simulink model "trimLiepke"  (R2021a)
settings: Solver=ode45  StartTime=0.0  StopTime=1000  RelTol=1e-3  EnableMultiTasking=on
undefined symbols (not defined in the file or in its folder): alpha_matrix, alphai, alt_matrix, b, beta, cbar, CD_0, CD_alpha, CD_de, CD_ih, CD_q, CL_0, Cl_0, CL_alpha, Cl_beta, Cl_da, CL_de, Cl_dr, CL_ih, Cl_p, CL_q, Cl_r, cla_matrix, clb_matrix, clp_matrix, clq_matrix, clr_matrix, Cm_0, Cm_alpha, Cm_de, Cm_ih, Cm_q, cma_matrix, cmq_matrix, Cn_0, Cn_beta, Cn_da, Cn_dr, Cn_p, Cn_r, cnb_matrix, cnp_matrix, cnr_matrix, CY_0, CY_beta, CY_da, CY_dr, CY_p, CY_r, cyb_matrix, cyp_matrix, H, Ix, Iy, Iz, Jxy, Jxz, Jyz, m, mach_matrix ... (+10)
libraries: airlib x3
(part 1 of 2)
settings Model: Creator=matt  LastModifiedBy=matt
settings SolverCC: AlgebraicLoopSolver=TrustRegion
settings DataIOCC: ExternalInput=[0 1 0 0 0 0 0 0 0 0 6.7015280237240514e-017]  InitialState=[100;0.33384643595852526;0;0;0;0;0;0.33384643595852531;0;0;0;60]  LoadExternalInput=on  LoadInitialState=on  SaveFormat=Array  SignalLoggingSaveFormat=ModelDataLogs  ReturnWorkspaceOutputs=off
settings OptimizationCC: BlockReduction=off  BooleanDataType=off
settings DebuggingCC: SaveWithParameterizedLinksMsg=none  UnderspecifiedInitializationDetection=Classic  MergeDetectMultiDrivingBlocksExec=none  SignalResolutionControl=TryResolveAllWithWarning  MultiTaskDSMMsg=warning  MultiTaskCondExecSysMsg=none  SFMachineParentedDataDiag=warning
settings HardwareCC: TargetUnknown=on
settings ModelReferenceCC: PropagateSignalLabelsOutOfModel=off
settings GRTTargetCC: CombineOutputUpdateFcns=off  GRTInterface=on

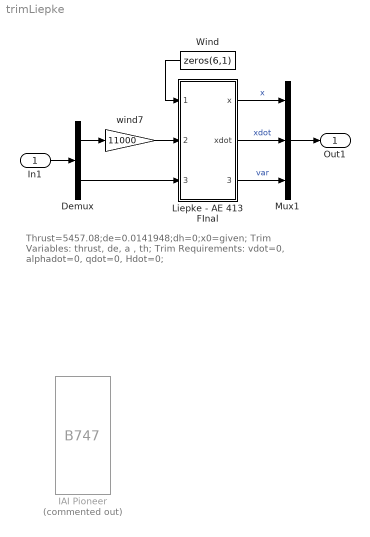
== system trimLiepke ==
  note: Thrust=5457.08;de=0.0141948;dh=0;x0=given;
      | Trim Variables: thrust, de, a , th;
      | Trim Requirements: vdot=0, alphadot=0, qdot=0, Hdot=0;
  In1 : Inport
  " IAI Pioneer " : airlib/B747  Commented=on  GM1="[0.5486  5.1511  2.8261   47.2259  90.9483  111.4754   0  -6.6462  0   190.512]"  CD_wind="[0.060  0.430  0  0.0180  0]"  CL_wind="[0.385  4.78  8.05  0.401  0]"  Cm_body="[0.194  -2.12   -36.6   -1.76    0]"  CY_body="[0   -0.819    0     0    0.191    0]"  Cl_body="[0   -0.023   -0.450   0.265   -0.161  -0.00229]"  Cn_body="[0    0.109  -0.110  -0.200    0.0200  -0.0917]"  x0="[60 -0.0293682 0   0 0 0   0 -0.0293682 0   0 0 60]"
  " Liepke - AE 413 FInal" : Subsystem  AncestorBlock=airlib/B747  mask(General Nonlinear Aircraft Model){GM1=[cbar   b   S   Ix  Iy  Iz   Jxy Jxz  Jyz   m], CD_wind=[CD_0   CD_alpha   CD_q   CD_de   CD_ih], CL_wind=[CL_0   CL_alpha   CL_q   CL_de   CL_ih], Cm_body=[Cm_0   Cm_alpha   Cm_q   Cm_de   Cm_ih], CY_body=[CY_0   CY_beta   CY_p   CY_r   CY_da   CY_dr], Cl_body=[Cl_0   Cl_beta   Cl_p   Cl_r   Cl_da   Cl_dr], Cn_body=[Cn_0   Cn_beta   Cn_p   Cn_r   Cn_da   Cn_dr], x0=[v alphai beta p q r psi theta phi xe ye H]}
      mask prompts: GM1 "Geometry and Mass : [cbar   b    S    Ix   Iy   Iz   Jxy  Jxz  Jyz  m]"; CD_wind "Aerodynamic D-Force Derivatives : [CD0 CDa CDq CDde CDih]"; CL_wind "Aerodynamic L-Force Derivatives : [CL0 CLa CLq CLde CLih]"; Cm_body "Aerodynamic Y-Moment Derivatives : [Cm0 Cma Cmq Cmde Cmih]"; CY_body "Aerodynamic Y-Force Derivatives : [CY0 CYb CYp CYr CYda CYdr]"; Cl_body "Aerodynamic X-moment Derivatives : [Cl0 Clb Clp Clr Clda Cldr]"; Cn_body "Aerodynamic Z-moment Derivatives : [Cn0 Cnb Cnp Cnr Cnda Cndr]"; x0 "Initial Condition x0 [v alpha beta p q r psi theta phi xe ye H]"
      mask help:
      | The first input contains the wind velocity and acceleration.
      |   The second input contains external forces and moments in body axis.
      |   The third input contains the deflections of elevators, ailerons, rudder,
      |   and flaps. For a list of outputs look under the mask.
      |   NB : The International measurement system (MKS) is adopted.
      mask init:
      | AM=zeros(6,19);
      | AM(1,[1 2 9 11 12])=reshape(CD_wind,1,5);
      | AM(3,[1 2 9 11 12])=reshape(CL_wind,1,5);
      | AM(5,[1 2 9 11 12])=reshape(Cm_body,1,5);
      | AM(2,[1 5 8 10 13 14])=reshape(CY_body,1,6);
      | AM(4,[1 5 8 10 13 14])=reshape(Cl_body,1,6);
      | AM(6,[1 5 8 10 13 14])=reshape(Cn_body,1,6);
      | 
      | Ix=GM1(4);Iy=GM1(5);Iz=GM1(6);
      | Jxy=GM1(7);Jxz=GM1(8);Jyz=GM1(9);
      | 
      | detI = Ix*Iy*Iz - 2*Jxy*Jxz*Jyz - Ix*Jyz^2 - Iy*Jxz^2 - Iz*Jxy^2;
      | I1   = Iy*Iz - Jyz^2;I2   = Jxy*Iz + Jyz*Jxz;
      | I3   = Jxy*Jyz + Iy*Jxz;I4   = Ix*Iz - Jxz^2;
      | I5   = Ix*Jyz + Jxy*Jxz;I6   = Ix*Iy - Jxy^2;
      | 
      | Pl  = I1/detI; Pm = I2/detI; Pn = I3/detI;
      | Ppp = -(Jxz*I2 - Jxy*I3)/detI;Ppq = (Jxz*I1 - Jyz*I2 - (Iy-Ix)*I3)/detI;
      | Ppr = -(Jxy*I1 + (Ix-Iz)*I2 - Jyz*I3)/detI;Pqq = (Jyz*I1 - Jxy*I3)/detI;
      | Pqr = -((Iz-Iy)*I1 - Jxy*I2 + Jxz*I3)/detI;Prr = -(Jyz*I1 - Jxz*I2)/detI;
      | 
      | Ql  = I2/detI; Qm = I4/detI; Qn = I5/detI;
      | Qpp = -(Jxz*I4 - Jxy*I5)/detI;Qpq = (Jxz*I2 - Jyz*I4 - (Iy-Ix)*I5)/detI;
      | Qpr = -(Jxy*I2 + (Ix-Iz)*I4 - Jyz*I5)/detI;Qqq = (Jyz*I2 - Jxy*I5)/detI;
      | Qqr = -((Iz-Iy)*I2 - Jxy*I4 + Jxz*I5)/detI;Qrr = -(Jyz*I2 - Jxz*I4)/detI;
      | 
      | Rl  = I3/detI; Rm = I5/detI; Rn = I6/detI;
      | Rpp = -(Jxz*I5 - Jxy*I6)/detI;
      | Rpq = (Jxz*I3 - Jyz*I5 - (Iy-Ix)*I6)/detI;
      | Rpr = -(Jxy*I3 + (Ix-Iz)*I5 - Jyz*I6)/detI;
      | Rqq = (Jyz*I3 - Jxy*I6)/detI;
      | Rqr = -((Iz-Iy)*I3 - Jxy*I5 + Jxz*I6)/detI;
      | Rrr = -(Jyz*I3 - Jxz*I5)/detI;
      | 
      | GM2 = [  Pl   Pm   Pn   Ppp  Ppq  Ppr  Pqq  Pqr  Prr ;
      |                Ql  Qm   Qn   Qpp  Qpq  Qpr  Qqq  Qqr  Qrr ;
      |                Rl  Rm   Rn   Rpp  Rpq  Rpr  Rqq  Rqr  Rrr ];
      | 
      | xfix=1;
      mask Help:
      | <p>
      | This block is a general nonlinear 6DOF aircraft model, with a very accurate built-in atmosphere model and constant aerodynamic derivatives.
      | The architecture of the block is largely based on the Aircraft block provided by the <A
      | HREF="http://www.mathworks.com/matlabcentral/fileexchange/loadFile.do?objectId=252&objectType=file">FDC toolbox</A> (Marc Rauw, 1993-2000).
      | </p>
      | <p>
      | The geometric and inertal data of the aircraft are entered as parameters in the first row of the mask. The other six rows contains the
      | non-dimensional aerodynamic derivatives. The last row is the initial state.
      | </p>
      | <p>
      | The first input contains the wind velocity and acceleration.
      | The second input contains external forces and moments in the aircraft body axis.
      | The third input contains the deflections of elevators, ailerons, rudder,
      | and flaps or stabilators. For a list of outputs look under the mask.
      | </p>
      | <p>
      | The control surface sign conventions are the same adopted in books such as Stevens-Lewis and Etkin, and in many flight simulators,
      | including the FDC toolbox. <br>
      | Specifically, positive elevator deflection causes negative pitching moment (Cmde &#60 0), positive rudder deflection causes negative yawing
      | moment (Cndr &#60 0), and positive aileron deflection causes negative rolling moment (Clda &#60 0). Another way to say the same thing is
      | that, the positive elevators deflection is Trailing Edge Down (TED), the positive rudder(s) deflection is Trailing Edge Left (TEL), and,
      | taking as TED the positive ailerons deflection, da=K*(da_right-da_left), with K usually equal to 1 (FDC) or 1/2.
      | </p>
      | <p>
      | Since this block is largely based on the FDC toolbox, i redirect you to the FDC Toolbox manual, for a good explanation of the underlying
      | components. Besides the mask and the fact that the aerodynamic derivatives are expressed in the stability axis, the only relevant difference
      | with the FDC toolbox is that in the computation of the aerodynamic forces, q is normalized as q*cbar/2V instead of q*cbar/V. The majority
      | of aeronautics books that i've seen use q*cbar/2V.
      | </p>
      | <p>
      | Please note that the International Measurement System is adopted. So, lengths are in meters, masses in Kg, and inertia moments in Kg*m^2.
      | Moreover, forces are in N, moments in N*m, accelerations in g, and angles in radians. For those that use the english system, here are some useful
      | conversion factors: <br>
      | 1 ft   = 0.3048 m, 1 lb   = 0.4536 Kg, 1 slug = 14.593903 Kg ,  1 slug*ft^2 = 1.355818 Kg*m^2
      | <br>
      | </p>
      | <p>
      | Finally, there is an <A HREF="http://www.aae.uiuc.edu/m-selig/apasim/Aircraft-uiuc.html">excellent source</A> of aircraft aerodynamic data
      | which is mantained by Michael S. Selig, Rob Deters, and Glen Dimock at the university of Urbana-Champaign. To use any of the given models
      | you just need to type the supplied aircraft data in the block mask.
      | </p>
      | <p>
      | <p>
      | December 2002, Giampiero Campa
      | </p>
      | </p>
      mask Display: disp('General\nAircraft\nModel')
  Demux : Demux  Outputs=[6 4]
      settings: DisplayOption=none
  Mux1 : Mux  Inputs=[12 12 12]
  Wind : Constant  Value=zeros(6,1)
  wind7 : Gain  Gain=11000  SaturateOnIntegerOverflow=on  OutDataTypeStr=Inherit: Same as input  ParamDataTypeStr=Inherit: Same as input
  Out1 : Outport
  wires:
  Demux/1 -> wind7/1
  In1/1 -> Demux/1
  Mux1/1 -> Out1/1
  Wind/1 -> " Liepke - AE 413 FInal"/1(" uwind")
  wind7/1 -> " Liepke - AE 413 FInal"/2(ext fm)
  Demux/2 -> " Liepke - AE 413 FInal"/3(deflect)
  " Liepke - AE 413 FInal"/1(x) -> Mux1/1  "x"
  " Liepke - AE 413 FInal"/2(xdot) -> Mux1/2  "xdot"
  " Liepke - AE 413 FInal"/3(others) -> Mux1/3  "var"

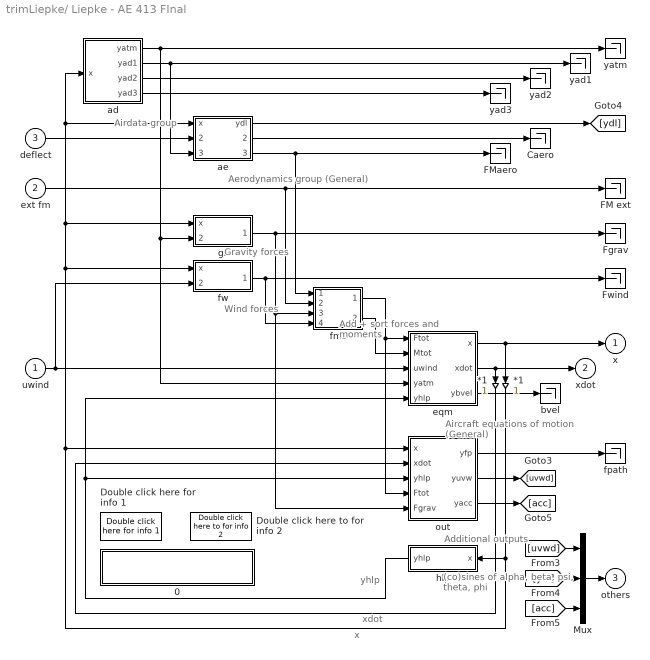
== system trimLiepke/ Liepke - AE 413 FInal ==
  note: xdot
  note: x
  note: yhlp
  note: Additional outputs
  note: Aircraft equations
      | of motion (General)
  note: Wind forces
  note: Gravity forces
  note: Aerodynamics
      | group (General)
  note: (co)sines of
      | alpha, beta,
      | psi, theta, phi
  note: Add + sort
      | forces and
      | moments
  note: Airdata group
  " uwind" : Inport
  ext fm : Inport  Port=2
  deflect : Inport  Port=3
  " *1" : Gain  SaturateOnIntegerOverflow=on  OutDataTypeStr=Inherit: Same as input  ParamDataTypeStr=Inherit: Same as input
  *1 : Gain  SaturateOnIntegerOverflow=on  OutDataTypeStr=Inherit: Same as input  ParamDataTypeStr=Inherit: Same as input
  0 : Subsystem
      mask Display: disp('AIRCRAFT, main level\nM.O. Rauw')
  Caero : Terminator
  Double click here for info 1 : airlib/DT-B747/Double click here for info 1  SystemSampleTime=-1  VariantActivationTime=update diagram  Latency=0  AutoFrameSizeCalculation=off
  Double click here to for info 2 : airlib/DT-B747/Double click here to for info 2  SystemSampleTime=-1  VariantActivationTime=update diagram  Latency=0  AutoFrameSizeCalculation=off
  FM ext : Terminator
  FMaero : Terminator
  Fgrav : Terminator
  Fwind : Terminator
  Mux : Mux  Inputs=[3 3 6]
  ad : Subsystem
  ae : Subsystem
  bvel : Terminator
  eqm : Subsystem
  fms : Subsystem  mask(FMsort){}
      mask help: Forces and Moments sorting block
      mask Display: disp('FMsort')
  fpath : Terminator
  fw : Subsystem  mask(fwind){m=GM1(10)}
      mask prompts: m "Mass of the aircraft [kg]:"
      mask help: Forces due to non-steady atmosphere.
      mask Display: disp('Fwind')
  gr : Subsystem  mask(Gravity){m=GM1(10)}
      mask prompts: m "Mass of the aircraft [kg]:"
      mask help: Gravity forces.
      mask Display: disp('Gravity')
  hlp : Subsystem  mask(Hlpfcn){}
      mask help: Help sines and cosines
      mask Display: disp('hlpfcn')
  out : Subsystem
  yad1 : Terminator
  yad2 : Terminator
  yad3 : Terminator
  yatm : Terminator
  x : Outport
  xdot : Outport  Port=2
  others : Outport  Port=3
  wires:
  fms/1(Ftot) -> out/4(Ftot), eqm/1(Ftot)
  ext fm/1 -> fms/2(FMprop), FM ext/1
  deflect/1 -> ae/2(uaero)
  ad/4(yad3) -> yad3/1
  ae/1(ydl) -> [ydl]
  ae/2(Caero) -> Caero/1
  eqm/3(ybvel) -> bvel/1
  out/1(yfp) -> fpath/1
  ad/2(yad1) -> ae/3(yad1), yad1/1
  ad/3(yad2) -> yad2/1
  ad/1(yatm) -> eqm/4(yatm), gr/2(yatm), yatm/1
  out/3(yacc) -> [acc]
  fw/1(Fwind) -> Fwind/1, fms/4(Fwind)
  ae/3(FMaero) -> FMaero/1, fms/1(FMaero)
  hlp/1(yhlp) -> eqm/5(yhlp), out/3(yhlp)
  " uwind"/1 -> eqm/3(uwind), fw/2(uwind)
  *1/1 -> out/2(xdot)
  gr/1(Fgrav) -> fms/3(Fgrav), out/5(Fgrav), Fgrav/1
  " *1"/1 -> hlp/1(x), out/1(x), fw/1(x), gr/1(x), ae/1(x), ad/1(x)
  eqm/2(xdot) -> xdot/1, *1/1
  eqm/1(x) -> x/1, " *1"/1
  fms/2(Mtot) -> eqm/2(Mtot)
  out/2(yuvw) -> [uvwd]
  [uvwd] -> Mux/1
  [ydl] -> Mux/2
  [acc] -> Mux/3
  Mux/1 -> others/1

== system trimLiepke/ Liepke - AE 413 FInal/0 ==

== system trimLiepke/ Liepke - AE 413 FInal/ad ==
  x : Inport
  0 : Subsystem
      mask Display: disp('AIRDATA GROUP (level 3)\nM.O. Rauw')
  ad1 : Subsystem  mask(Airdata1){}
      mask help: Basic airdata variables
      mask Display: disp('Airdata1')
  ad2 : Subsystem  mask(Airdata2){}
      mask help: More airdata variables
      mask Display: disp('Airdata2')
  ad3 : Subsystem  mask(Airdata3){cbar=GM1(1)}
      mask prompts: cbar "Mean aerodynamic chord [m]:"
      mask help: More airdata variables
      mask Display: disp('Airdata3')
  atm : Subsystem  mask(Atmosph){}
      mask help: Atmosphere variables
      mask Display: disp('Atmosph')
  yatm : Outport
  yad1 : Outport  Port=2
  yad2 : Outport  Port=3
  yad3 : Outport  Port=4
  wires:
  ad2/1(yad2) -> yad2/1
  ad3/1(yad3) -> yad3/1
  x/1 -> atm/1(x), ad1/1(x), ad3/1(x)
  atm/1(yatm) -> yatm/1, ad1/2(yatm), ad2/1(yatm), ad3/2(yatm)
  ad1/1(yad1) -> yad1/1, ad2/2(yad1), ad3/3(yad1)

== system trimLiepke/ Liepke - AE 413 FInal/ae ==
  x : Inport
  uaero : Inport  Port=2
  yad1 : Inport  Port=3
  0 : Subsystem
      mask Display: disp('AERODYNAMICS GROUP (level 3)\nM.O. Rauw')
  aero : Subsystem  mask(Aeromod){}
      mask help: Aerodynamic model of the DHC-2 'Beaver'.
      mask Display: disp('Aeromod\n(General)')
  dl : Subsystem  mask(Dimless){cbar=GM1(1), b=GM1(2)}
      mask prompts: cbar "Mean aerodynamic chord [m]:"; b "Wing span [m]:"
      mask help: Dimensionless rotational velocities.
      mask Display: disp('Dimless')
  fmdims : Subsystem  mask(FMdims){cbar=GM1(1), b=GM1(2), S=GM1(3)}
      mask prompts: cbar "Mean aerodynamic chord [m]:"; b "Wing span [m]:"; S "Wing surface [m^2]:"
      mask help:
      | Calculate forces and moments from
      | dimensionless derivatives.
      mask Display: disp('FMdims')
  ydl : Outport
  Caero : Outport  Port=2
  FMaero : Outport  Port=3
  wires:
  aero/1(Caero) -> Caero/1, fmdims/2(Force / moment derivatives)
  dl/1(ydl) -> aero/3(ydl), ydl/1
  x/1 -> aero/1(x), dl/1(x)
  uaero/1 -> aero/2(uaero)
  yad1/1 -> aero/4(Input), fmdims/1(yad1)
  fmdims/1(Forces and moments) -> FMaero/1

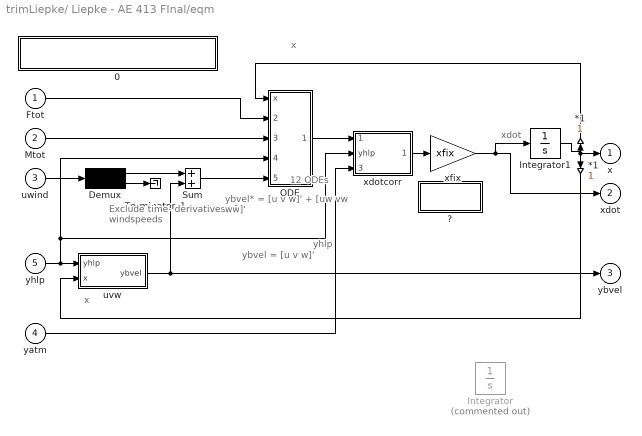
== system trimLiepke/ Liepke - AE 413 FInal/eqm ==
  note: Exclude time-
      | derivatives
      | of windspeeds
  note: ybvel* =
      | [u v w]' +
      | [uw vw ww]'
  note: xdot
  note: x
  note: x
  note: yhlp
  note: ybvel = [u v w]'
  note: 12 ODEs
  Ftot : Inport
  Mtot : Inport  Port=2
  uwind : Inport  Port=3
  yatm : Inport  Port=4
  yhlp : Inport  Port=5
  " *1" : Gain  SaturateOnIntegerOverflow=on  OutDataTypeStr=Inherit: Same as input  ParamDataTypeStr=Inherit: Same as input
  *1 : Gain  SaturateOnIntegerOverflow=on  OutDataTypeStr=Inherit: Same as input  ParamDataTypeStr=Inherit: Same as input
  0 : Subsystem
      mask Display: disp('EQUATIONS OF MOTION (level 3)\nM.O. Rauw')
  "?" : Subsystem
      mask Display: disp('More info\nfor xfix')
  Demux : Demux  Outputs=[3 3]
      settings: DisplayOption=none
  Integrator : Integrator  Commented=on  InitialCondition=x0
  Integrator1 : Integrator  InitialCondition=x0
  ODE : Subsystem
  Sum : Sum  InputSameDT=on  SaturateOnIntegerOverflow=on  OutDataTypeStr=Inherit: Same as first input
  Terminator_1 : Terminator
  uvw : Subsystem  mask(uvw){}
      mask help:
      | Calculation of body-axes velocities
      | u, v, and w
      mask Display: disp('Body-axes\nvelocities')
  xdotcorr : Subsystem  mask(xdotcorr){b=GM1(2), S=GM1(3), m=GM1(10), CYbdot=AM(2,19)}
      mask prompts: b "Wing span [m]:"; S "Wing surface [m^2]:"; m "Mass of the aircraft [kg]:"; CYbdot "Stability-derivative CYbdot:"
      mask help:
      | Correction block to write state
      | equations for DHC-2 Beaver aircraft
      | explicitly.
      mask Display: disp('xdotcorr\n(General)')
  xfix : Gain  Gain=xfix  SaturateOnIntegerOverflow=on  OutDataTypeStr=Inherit: Same as input  ParamDataTypeStr=Inherit: Same as input
  x : Outport
  xdot : Outport  Port=2
  ybvel : Outport  Port=3
  wires:
  Demux/2 -> Terminator_1/1
  yhlp/1 -> uvw/1(yhlp), ODE/4(yhlp), xdotcorr/2(yhlp)
  ODE/1(xdot) -> xdotcorr/1(xdot uncorrected)
  Sum/1 -> ODE/5(ybvel*)
  uvw/1(ybvel) -> ybvel/1, Sum/2
  uwind/1 -> Demux/1
  Demux/1 -> Sum/1
  xdotcorr/1(xdot corrected) -> xfix/1
  yatm/1 -> xdotcorr/3(yatm)
  Ftot/1 -> ODE/2(Ftot)
  Mtot/1 -> ODE/3(Mtot)
  *1/1 -> uvw/2(x)
  Integrator1/1 -> x/1, " *1"/1, *1/1
  xfix/1 -> Integrator1/1, xdot/1
  " *1"/1 -> ODE/1(x)

== system trimLiepke/ Liepke - AE 413 FInal/fms ==
  FMaero : Inport
  FMprop : Inport  Port=2
  Fgrav : Inport  Port=3
  Fwind : Inport  Port=4
  0 : Subsystem
      mask Display: disp('FMSORT\nM.O. Rauw, October 1997')
  Demux : Demux  Outputs=[3 3]
      settings: DisplayOption=none
  Demux1 : Demux  Outputs=[3 3]
      settings: DisplayOption=none
  Sum1 : Sum  InputSameDT=on  SaturateOnIntegerOverflow=on  OutDataTypeStr=Inherit: Same as first input
  Sum3 : Sum  Inputs=++++  InputSameDT=on  SaturateOnIntegerOverflow=on  OutDataTypeStr=Inherit: Same as first input
  Ftot : Outport
  Mtot : Outport  Port=2
  wires:
  FMaero/1 -> Demux/1
  FMprop/1 -> Demux1/1
  Demux1/2 -> Sum1/2
  Demux/2 -> Sum1/1
  Fgrav/1 -> Sum3/3
  Demux1/1 -> Sum3/2
  Sum3/1 -> Ftot/1
  Sum1/1 -> Mtot/1
  Demux/1 -> Sum3/1
  Fwind/1 -> Sum3/4

== system trimLiepke/ Liepke - AE 413 FInal/fw ==
  x : Inport
  uwind : Inport  Port=2
  -Xw/m : Fcn  Expr=u[16] + u[5]*u[15] - u[6]*u[14]
  -Yw/m : Fcn  Expr=u[17] - u[4]*u[15] + u[6]*u[13]
  -Zw/m : Fcn  Expr=u[18] + u[4]*u[14] - u[5]*u[13]
  0 : Subsystem
      mask Display: disp('FWIND\nM.O. Rauw, Dec. 1996')
  Mux : Mux  Inputs=3
  Mux1 : Mux  Inputs=[12 6]
  gain : Gain  Gain=-m  SaturateOnIntegerOverflow=on  OutDataTypeStr=Inherit: Same as input  ParamDataTypeStr=Inherit: Same as input
  Fwind : Outport
  wires:
  uwind/1 -> Mux1/2
  x/1 -> Mux1/1
  gain/1 -> Fwind/1
  Mux/1 -> gain/1
  Mux1/1 -> -Yw/m/1, -Zw/m/1, -Xw/m/1
  -Yw/m/1 -> Mux/2
  -Xw/m/1 -> Mux/1
  -Zw/m/1 -> Mux/3

== system trimLiepke/ Liepke - AE 413 FInal/gr ==
  x : Inport
  yatm : Inport  Port=2
  0 : Subsystem
      mask Display: disp('GRAVITY\nM.O. Rauw, October 1997')
  Mux : Mux  Inputs=3
  Mux1 : Mux  Inputs=[12 5]
  Xgr : Fcn  Expr=-m*u[17]*sin(u[8])
  Ygr : Fcn  Expr=m*u[17]*cos(u[8])*sin(u[9])
  Zgr : Fcn  Expr=m*u[17]*cos(u[8])*cos(u[9])
  Fgrav : Outport
  wires:
  Xgr/1 -> Mux/1
  Ygr/1 -> Mux/2
  Mux/1 -> Fgrav/1
  Mux1/1 -> Ygr/1, Xgr/1, Zgr/1
  Zgr/1 -> Mux/3
  x/1 -> Mux1/1
  yatm/1 -> Mux1/2

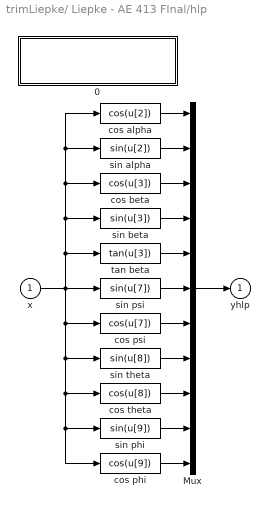
== system trimLiepke/ Liepke - AE 413 FInal/hlp ==
  x : Inport
  0 : Subsystem
      mask Display: disp('HELP FUNCTIONS\n(often used sines and cosines)\nM.O. Rauw, October 1997')
  Mux : Mux  Inputs=11
  cos alpha : Fcn  Expr=cos(u[2])
  cos beta : Fcn  Expr=cos(u[3])
  cos phi : Fcn  Expr=cos(u[9])
  cos psi : Fcn  Expr=cos(u[7])
  cos theta : Fcn  Expr=cos(u[8])
  sin alpha : Fcn  Expr=sin(u[2])
  sin beta : Fcn  Expr=sin(u[3])
  sin phi : Fcn  Expr=sin(u[9])
  sin psi : Fcn  Expr=sin(u[7])
  sin theta : Fcn  Expr=sin(u[8])
  tan beta : Fcn  Expr=tan(u[3])
  yhlp : Outport
  wires:
  x/1 -> sin psi/1, sin beta/1, cos beta/1, sin alpha/1, cos alpha/1, tan beta/1, sin theta/1, cos theta/1, sin phi/1, cos phi/1, cos psi/1
  cos alpha/1 -> Mux/1
  sin alpha/1 -> Mux/2
  cos beta/1 -> Mux/3
  sin beta/1 -> Mux/4
  tan beta/1 -> Mux/5
  sin psi/1 -> Mux/6
  cos psi/1 -> Mux/7
  sin theta/1 -> Mux/8
  cos theta/1 -> Mux/9
  sin phi/1 -> Mux/10
  Mux/1 -> yhlp/1
  cos phi/1 -> Mux/11

== system trimLiepke/ Liepke - AE 413 FInal/out ==
  note: Flightpath
      | variables
  note: du/dt, dv/dt, dw/dt
      | (output equations!)
  note: Body-axes accelerations
      | and specific forces
  x : Inport
  xdot : Inport  Port=2
  yhlp : Inport  Port=3
  Ftot : Inport  Port=4
  Fgrav : Inport  Port=5
  0 : Subsystem
      mask Display: disp('Additional outputs (level 3)\nM.O. Rauw')
  accel : Subsystem  mask(accel){m=GM1(10)}
      mask prompts: m "Mass of the aircraft [kg]:"
      mask help:
      | Body axes accelerations and
      | specific forces.
      mask Display: disp('Accel')
  fp : Subsystem  mask(Flpath){alpha0=x0(2)}
      mask prompts: alpha0 "Initial value of angle of attack, alpha0:"
      mask help: Flightpath related parameters.
      mask Display: disp('flpath')
  uvwdot : Subsystem  mask(uvwdot){}
      mask help: Calculation of du/dt, dv/dt, and dw/dt.
      mask Display: disp('uvwdot')
  yfp : Outport
  yuvw : Outport  Port=2
  yacc : Outport  Port=3
  wires:
  fp/1(yfp) -> yfp/1
  uvwdot/1(yuvw = [udot; vdot; wdot]) -> yuvw/1
  yhlp/1 -> uvwdot/3(yhlp)
  Ftot/1 -> accel/1(Ftot)
  accel/1(yacc) -> yacc/1
  xdot/1 -> fp/2(xdot), uvwdot/2(xdot)
  x/1 -> fp/1(x), uvwdot/1(x)
  Fgrav/1 -> accel/2(Fgrav)

== system trimLiepke/ Liepke - AE 413 FInal/ad/0 ==

== system trimLiepke/ Liepke - AE 413 FInal/ad/ad1 ==
  x : Inport
  yatm : Inport  Port=2
  0 : Subsystem
      mask Display: disp('AIRDATA1\nM.O. Rauw, October 1997')
  M : Fcn  Expr=u[2]/u[1]
  Mux : Mux  Inputs=[1 12]
  Mux1 : Mux  Inputs=[12 5]
  Mux2 : Mux  Inputs=3
  a : Fcn  Expr=sqrt(401.8743*u[3])
  qdyn : Fcn  Expr=0.5*u[13]*u[1]^2
  yad1 : Outport
  wires:
  Mux2/1 -> yad1/1
  qdyn/1 -> Mux2/3
  a/1 -> Mux/1, Mux2/1
  M/1 -> Mux2/2
  Mux1/1 -> qdyn/1
  Mux/1 -> M/1
  x/1 -> Mux/2, Mux1/1
  yatm/1 -> a/1, Mux1/2

== system trimLiepke/ Liepke - AE 413 FInal/ad/ad2 ==
  yatm : Inport
  yad1 : Inport  Port=2
  0 : Subsystem
      mask Display: disp('AIRDATA2\nM.O. Rauw, October 1997')
  Mux : Mux  Inputs=[5 3]
  Mux1 : Mux  Inputs=3
  Vc : Fcn  Expr=sqrt(579000*((1+u[1]/101325)^(1/3.5)-1))
  Ve : Fcn  Expr=sqrt(u[8] * 1.63265)
  qc : Fcn  Expr=u[2] * ((1+0.2*u[7]^2)^3.5-1)
  yad2 : Outport
  wires:
  yad1/1 -> Mux/2
  yatm/1 -> Mux/1
  Mux/1 -> qc/1, Ve/1
  Ve/1 -> Mux1/2
  Vc/1 -> Mux1/3
  qc/1 -> Vc/1, Mux1/1
  Mux1/1 -> yad2/1

== system trimLiepke/ Liepke - AE 413 FInal/ad/ad3 ==
  x : Inport
  yatm : Inport  Port=2
  yad1 : Inport  Port=3
  0 : Subsystem
      mask Display: disp('AIRDATA3\nM.O. Rauw, October 1997')
  Mux : Mux  Inputs=3
  Mux1 : Mux  Inputs=[12 5 3]
  Re : Fcn  Expr=(u[13]*u[1])/u[16]
  Tt : Fcn  Expr=u[15] * (1+0.2*u[19]^2)
  cbar : Gain  Gain=cbar  SaturateOnIntegerOverflow=on  OutDataTypeStr=Inherit: Same as input  ParamDataTypeStr=Inherit: Same as input
  yad3 : Outport
  wires:
  yad1/1 -> Mux1/3
  yatm/1 -> Mux1/2
  x/1 -> Mux1/1
  Re/1 -> Mux/2, cbar/1
  Mux1/1 -> Re/1, Tt/1
  Mux/1 -> yad3/1
  Tt/1 -> Mux/1
  cbar/1 -> Mux/3

== system trimLiepke/ Liepke - AE 413 FInal/ad/atm ==
  x : Inport
  0 : Subsystem
      mask Display: disp('ATMOSPH\nM.O. Rauw, October 1997')
  Mux : Mux  Inputs=2
  Mux1 : Mux  Inputs=[2 1]
  Mux2 : Mux  Inputs=5
  T : Fcn  Expr=288.15 - 0.0065*u[12]
  g : Fcn  Expr=9.80665*(6371020/(6371020+u[12]))^2
  mu : Fcn  Expr=(1.458*10^(-6)*u[2]^1.5)/(u[2]+110.4)
  ps : Fcn  Expr=101325*(u[2]/288.15)^(u[1]/1.86584)
  rho : Fcn  Expr=u[3]/(287.053*u[2])
  yatm : Outport
  wires:
  x/1 -> T/1, g/1
  Mux/1 -> Mux1/1, mu/1, ps/1
  ps/1 -> Mux1/2, Mux2/2
  T/1 -> Mux/2, Mux2/3
  g/1 -> Mux/1, Mux2/5
  rho/1 -> Mux2/1
  Mux1/1 -> rho/1
  Mux2/1 -> yatm/1
  mu/1 -> Mux2/4

== system trimLiepke/ Liepke - AE 413 FInal/ae/0 ==

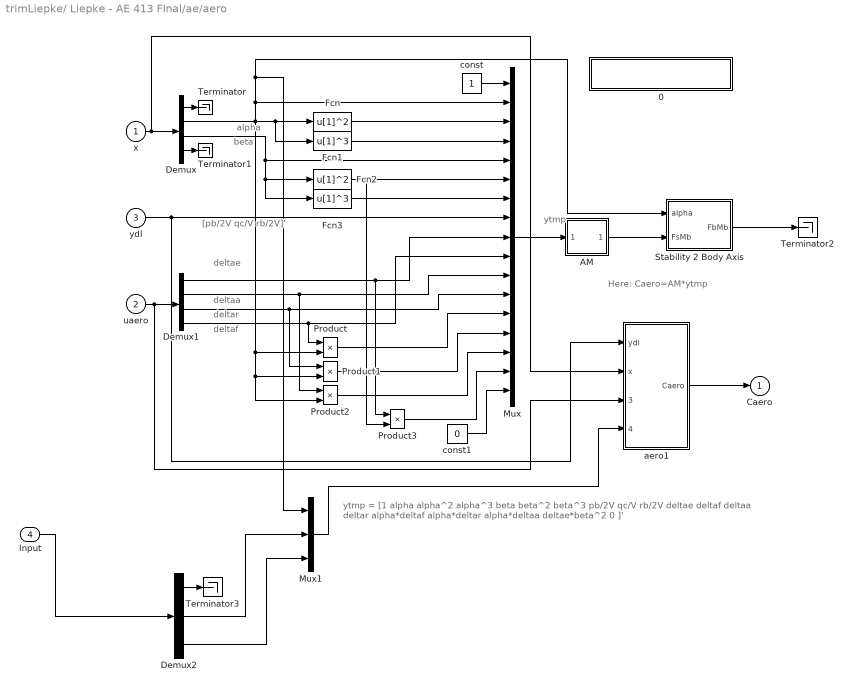
== system trimLiepke/ Liepke - AE 413 FInal/ae/aero ==
  note: [pb/2V qc/V rb/2V]'
  note: beta
  note: deltaf
  note: ytmp = [1  alpha  alpha^2  alpha^3  beta  beta^2  beta^3  pb/2V  qc/V  rb/2V  deltae
      | deltaf  deltaa  deltar  alpha*deltaf  alpha*deltar  alpha*deltaa  deltae*beta^2  0 ]'
  note: deltaa
  note: deltae
  note: deltar
  note: alpha
  note: ytmp
  note: Here: Caero=AM*ytmp
  x : Inport
  uaero : Inport  Port=2
  ydl : Inport  Port=3
  Input : Inport  Port=4
  0 : Subsystem
      mask Display: disp('AEROMOD\nM.O. Rauw, October 1997')
  "AM " : Subsystem  mask(State Space){M=AM}
      mask prompts: M "Matrix"
      mask Display: disp('Matrix\nGain')
  Demux : Demux  Outputs=[1 1 1 9]
      settings: DisplayOption=none
  Demux1 : Demux
      settings: DisplayOption=none
  Demux2 : Demux  Outputs=3
  Fcn : Fcn  Expr=u[1]^2
  Fcn1 : Fcn  Expr=u[1]^3
  Fcn2 : Fcn  Expr=u[1]^2
  Fcn3 : Fcn  Expr=u[1]^3
  Mux : Mux  Inputs=[1 1 1 1 1 1 1 3 1 1 1 1 1 1 1 1 1]
  Mux1 : Mux  Inputs=3
  Product{,1..3} (4 alike) : Product  InputSameDT=on  RndMeth=Zero  SaturateOnIntegerOverflow=on  OutDataTypeStr=Inherit: Same as first input
  Stability 2 Body Axis : Subsystem
  Terminator{,1..3} (4 alike) : Terminator
  aero1 : Subsystem
      mask Display: disp('Derivatives')
  const : Constant
  const1 : Constant  Value=0
  Caero : Outport  VectorParamsAs1DForOutWhenUnconnected=off
  wires:
  ydl/1 -> aero1/1(ydl), Mux/8
  "AM "/1(Out1) -> Stability 2 Body Axis/2(FsMb)
  Stability 2 Body Axis/1(FbMb) -> Terminator2/1
  Fcn/1 -> Mux/3
  Mux/1 -> "AM "/1(In1)
  Demux/2 -> Fcn/1, Fcn1/1, Product/2, Product1/2, Product2/2, Mux/2, Mux1/1, Stability 2 Body Axis/1(alpha)
  x/1 -> aero1/2(x), Demux/1
  Fcn3/1 -> Mux/7
  Demux1/2 -> Mux/11, Product2/1
  Product2/1 -> Mux/15
  const1/1 -> Mux/17
  Fcn1/1 -> Mux/4
  Demux/1 -> Terminator/1
  aero1/1(Caero) -> Caero/1
  uaero/1 -> aero1/3(Controls), Demux1/1
  Product3/1 -> Mux/16
  Demux1/4 -> Mux/10, Product/1
  Fcn2/1 -> Mux/6, Product3/2
  Demux/3 -> Mux/5, Fcn2/1, Fcn3/1
  Demux1/1 -> Mux/9, Product3/1
  Product1/1 -> Mux/14
  const/1 -> Mux/1
  Demux1/3 -> Mux/12, Product1/1
  Demux/4 -> Terminator1/1
  Product/1 -> Mux/13
  Input/1 -> Demux2/1
  Demux2/2 -> Mux1/2
  Demux2/3 -> Mux1/3
  Mux1/1 -> aero1/4("[alpha,mach,alt]")
  Demux2/1 -> Terminator3/1

== system trimLiepke/ Liepke - AE 413 FInal/ae/dl ==
  x : Inport
  0 : Subsystem
      mask Display: disp('DIMLESS\nM.O. Rauw, October 1997')
  Mux : Mux  Inputs=3
  pb/2V : Fcn  Expr=0.5 * u[4] * b / u[1]
  qc/2V : Fcn  Expr=0.5* u[5] * cbar / u[1]
  rb/2V : Fcn  Expr=0.5 * u[6] * b / u[1]
  ydl : Outport
  wires:
  pb/2V/1 -> Mux/1
  qc/2V/1 -> Mux/2
  rb/2V/1 -> Mux/3
  Mux/1 -> ydl/1
  x/1 -> qc/2V/1, rb/2V/1, pb/2V/1

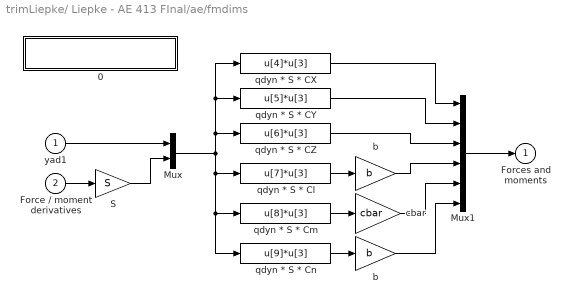
== system trimLiepke/ Liepke - AE 413 FInal/ae/fmdims ==
  yad1 : Inport
  Force / moment derivatives : Inport  Port=2
  0 : Subsystem
      mask Display: disp('FMDIMS\nM.O. Rauw, October 1997')
  Mux : Mux  Inputs=[3 6]
  Mux1 : Mux  Inputs=6
  S : Gain  Gain=S  SaturateOnIntegerOverflow=on  OutDataTypeStr=Inherit: Same as input  ParamDataTypeStr=Inherit: Same as input
  b : Gain  Gain=b  SaturateOnIntegerOverflow=on  OutDataTypeStr=Inherit: Same as input  ParamDataTypeStr=Inherit: Same as input
  "b " : Gain  Gain=b  SaturateOnIntegerOverflow=on  OutDataTypeStr=Inherit: Same as input  ParamDataTypeStr=Inherit: Same as input
  cbar : Gain  Gain=cbar  SaturateOnIntegerOverflow=on  OutDataTypeStr=Inherit: Same as input  ParamDataTypeStr=Inherit: Same as input
  qdyn * S * CX : Fcn  Expr=u[4]*u[3]
  qdyn * S * CY : Fcn  Expr=u[5]*u[3]
  qdyn * S * CZ : Fcn  Expr=u[6]*u[3]
  qdyn * S * Cl : Fcn  Expr=u[7]*u[3]
  qdyn * S * Cm : Fcn  Expr=u[8]*u[3]
  qdyn * S * Cn : Fcn  Expr=u[9]*u[3]
  Forces and moments : Outport
  wires:
  Mux1/1 -> Forces and moments/1
  "b "/1 -> Mux1/6
  cbar/1 -> Mux1/5
  Force / moment derivatives/1 -> S/1
  Mux/1 -> qdyn * S * CZ/1, qdyn * S * CX/1, qdyn * S * CY/1, qdyn * S * Cl/1, qdyn * S * Cm/1, qdyn * S * Cn/1
  qdyn * S * Cl/1 -> b/1
  qdyn * S * Cm/1 -> cbar/1
  qdyn * S * Cn/1 -> "b "/1
  yad1/1 -> Mux/1
  qdyn * S * CX/1 -> Mux1/1
  qdyn * S * CY/1 -> Mux1/2
  S/1 -> Mux/2
  qdyn * S * CZ/1 -> Mux1/3
  b/1 -> Mux1/4

== system trimLiepke/ Liepke - AE 413 FInal/eqm/0 ==

== system trimLiepke/ Liepke - AE 413 FInal/eqm/? ==

== system trimLiepke/ Liepke - AE 413 FInal/eqm/ODE ==
  x : Inport
  Ftot : Inport  Port=2
  Mtot : Inport  Port=3
  yhlp : Inport  Port=4
  ybvel* : Inport  Port=5
  0 : Subsystem
      mask Display: disp('12 Ordinary Differential\nEquations (level 4)\nM.O. Rauw')
  Eulerdot : Subsystem  mask(Eulerdot){}
      mask help:
      | Calculation of d(psi)/dt, d(theta)/dt,
      | and d(phi/dt)
      mask Display: disp('psi dot\ntheta dot\nphi dot')
  Mux : Mux  Inputs=[12 3 3 11]
  Mux1 : Mux  Inputs=[3 3 3 3]
  Vabdot : Subsystem  mask(Vabdot){m=GM1(10)}
      mask prompts: m "Mass of the aircraft [kg]:"
      mask help: Calculation of dV/dt, dalpha/dt, dbeta/dt.
      mask Display: disp('V dot\nalpha dot\nbeta dot')
  pqrdot : Subsystem  mask(pqrdot){}
      mask help: Calculation of dp/dt, dq/dt, and dr/dt
      mask Display: disp('p dot\nq dot\nr dot')
  xyHdot : Subsystem  mask(xyHdot){}
      mask help: Calculation of d(xe)/dt, d(ye)/dt, and dH/dt
      mask Display: disp('xe dot\nye dot\nH dot')
  xdot : Outport
  wires:
  x/1 -> Mux/1
  Mtot/1 -> Mux/3
  Ftot/1 -> Mux/2
  Mux/1 -> pqrdot/1(upqr), Vabdot/1(uVab), Eulerdot/1(ueul), xyHdot/2(uxYH)
  ybvel*/1 -> xyHdot/1(ybvel*)
  yhlp/1 -> Mux/4
  xyHdot/1(yxyH) -> Mux1/4
  Eulerdot/1(yeul) -> Mux1/3
  pqrdot/1(ypqr) -> Mux1/2
  Vabdot/1(yVab) -> Mux1/1
  Mux1/1 -> xdot/1

== system trimLiepke/ Liepke - AE 413 FInal/eqm/uvw ==
  yhlp : Inport
  x : Inport  Port=2
  0 : Subsystem
      mask Display: disp('UVW\nM.O. Rauw, October 1997')
  Mux : Mux  Inputs=3
  Mux1 : Mux  Inputs=[12 11]
  u : Fcn  Expr=u[1]*u[13]*u[15]
  v : Fcn  Expr=u[1]*u[16]
  w : Fcn  Expr=u[1]*u[14]*u[15]
  ybvel : Outport
  wires:
  Mux1/1 -> v/1, u/1, w/1
  yhlp/1 -> Mux1/2
  x/1 -> Mux1/1
  u/1 -> Mux/1
  v/1 -> Mux/2
  w/1 -> Mux/3
  Mux/1 -> ybvel/1

== system trimLiepke/ Liepke - AE 413 FInal/eqm/xdotcorr ==
  xdot uncorrected : Inport
  yhlp : Inport  Port=2
  yatm : Inport  Port=3
  0 : Subsystem
      mask Display: disp('XDOTCORR (General)\nM.O. Rauw, October 1997')
  Demux : Demux  Outputs=12
      settings: DisplayOption=none
  Mux1 : Mux  Inputs=12
  Mux2 : Mux  Inputs=[11 1 5]
  beta dot correction : Fcn  Expr=u[12] / (1 - (u[3]*u[13]*b*S*CYbdot)/(4*m))
  xdot corrected : Outport
  wires:
  beta dot correction/1 -> Mux1/3
  yatm/1 -> Mux2/3
  Demux/1 -> Mux1/1
  Demux/2 -> Mux1/2
  Demux/4 -> Mux1/4
  Demux/5 -> Mux1/5
  Demux/6 -> Mux1/6
  Demux/7 -> Mux1/7
  Demux/8 -> Mux1/8
  Demux/9 -> Mux1/9
  Demux/10 -> Mux1/10
  Demux/11 -> Mux1/11
  Demux/12 -> Mux1/12
  Demux/3 -> Mux2/2
  xdot uncorrected/1 -> Demux/1
  Mux1/1 -> xdot corrected/1
  Mux2/1 -> beta dot correction/1
  yhlp/1 -> Mux2/1

== system trimLiepke/ Liepke - AE 413 FInal/fms/0 ==

== system trimLiepke/ Liepke - AE 413 FInal/fw/0 ==

== system trimLiepke/ Liepke - AE 413 FInal/gr/0 ==

== system trimLiepke/ Liepke - AE 413 FInal/hlp/0 ==

== system trimLiepke/ Liepke - AE 413 FInal/out/0 ==

== system trimLiepke/ Liepke - AE 413 FInal/out/accel ==
  Ftot : Inport
  Fgrav : Inport  Port=2
  0 : Subsystem
      mask Display: disp('ACCEL\nM.O. Rauw, October 1997')
  Ax : Fcn  Expr=(u[1]-u[4])/(m*9.80665)
  Ay : Fcn  Expr=(u[2]-u[5])/(m*9.80665)
  Az : Fcn  Expr=(u[3]-u[6])/(m*9.80665)
  Mux : Mux  Inputs=6
  Mux1 : Mux  Inputs=[3 3]
  axk : Fcn  Expr=u[1]/(m*9.80665)
  ayk : Fcn  Expr=u[2]/(m*9.80665)
  azk : Fcn  Expr=u[3]/(m*9.80665)
  yacc : Outport
  wires:
  Ftot/1 -> Mux1/1
  Fgrav/1 -> Mux1/2
  Mux/1 -> yacc/1
  azk/1 -> Mux/6
  Az/1 -> Mux/3
  Ay/1 -> Mux/2
  Ax/1 -> Mux/1
  Mux1/1 -> Az/1, Ax/1, Ay/1, axk/1, azk/1, ayk/1
  axk/1 -> Mux/4
  ayk/1 -> Mux/5

== system trimLiepke/ Liepke - AE 413 FInal/out/fp ==
  x : Inport
  xdot : Inport  Port=2
  0 : Subsystem
      mask Display: disp('FLPATH\nM.O. Rauw, October 1997')
  Mux : Mux  Inputs=[12 12]
  Mux1 : Mux
  Phi : Fcn  Expr=u[9]*cos(u[8]-alpha0)
  chi : Fcn  Expr=u[3]+u[7]
  fpa : Fcn  Expr=u[13]/9.80665
  gamma : Fcn  Expr=asin(u[24]/u[1])
  yfp : Outport
  wires:
  gamma/1 -> Mux1/1
  Mux/1 -> chi/1, Phi/1, fpa/1, gamma/1
  fpa/1 -> Mux1/2
  chi/1 -> Mux1/3
  Phi/1 -> Mux1/4
  Mux1/1 -> yfp/1
  x/1 -> Mux/1
  xdot/1 -> Mux/2

== system trimLiepke/ Liepke - AE 413 FInal/out/uvwdot ==
  note: `
  note: cos(alpha)
  note: sin(alpha)
  note: cos(beta)
  note: sin(beta)
  note: V
  x : Inport
  xdot : Inport  Port=2
  yhlp : Inport  Port=3
  0 : Subsystem
      mask Display: disp('UVWDOT\nM.O. Rauw, October 1997')
  DeMux : Demux  Outputs=[1 1 1 1 7]
      settings: DisplayOption=none
  Demux : Demux  Outputs=[1 11]
      settings: DisplayOption=none
  Mux : Mux  Inputs=[1 1 1 1 1 12]
  Mux1 : Mux  Inputs=3
  Terminator : Terminator
  Terminator1 : Terminator
  u dot : Fcn  Expr=u[6]*u[1]*u[3] - u[5]*(u[7]*u[2]*u[3] + u[8]*u[1]*u[4])
  v dot : Fcn  Expr=u[6]*u[4] + u[5]*u[3]*u[8]
  wdot : Fcn  Expr=u[6]*u[2]*u[3] + u[5]*(u[7]*u[1]*u[3] - u[8]*u[2]*u[4])
  yuvw = [udot; vdot; wdot] : Outport
  wires:
  Demux/2 -> Terminator1/1
  DeMux/5 -> Terminator/1
  wdot/1 -> Mux1/3
  v dot/1 -> Mux1/2
  u dot/1 -> Mux1/1
  xdot/1 -> Mux/6
  Mux/1 -> v dot/1, wdot/1, u dot/1
  DeMux/1 -> Mux/1
  DeMux/2 -> Mux/2
  x/1 -> Demux/1
  Mux1/1 -> yuvw = [udot; vdot; wdot]/1
  yhlp/1 -> DeMux/1
  DeMux/3 -> Mux/3
  DeMux/4 -> Mux/4
  Demux/1 -> Mux/5

== system trimLiepke/ Liepke - AE 413 FInal/ad/ad1/0 ==

== system trimLiepke/ Liepke - AE 413 FInal/ad/ad2/0 ==

== system trimLiepke/ Liepke - AE 413 FInal/ad/ad3/0 ==

== system trimLiepke/ Liepke - AE 413 FInal/ad/atm/0 ==

== system trimLiepke/ Liepke - AE 413 FInal/ae/aero/0 ==

== system trimLiepke/ Liepke - AE 413 FInal/ae/aero/AM  ==
  In1 : Inport
  Matrix Gain : StateSpace  A=[]  B=[]  C=[]  D=M  InitialCondition=0
  Out1 : Outport  VectorParamsAs1DForOutWhenUnconnected=off
  wires:
  In1/1 -> Matrix Gain/1
  Matrix Gain/1 -> Out1/1

== system trimLiepke/ Liepke - AE 413 FInal/ae/aero/Stability 2 Body Axis ==
  alpha : Inport
  FsMb : Inport  Port=2
  Demux2 : Demux  Outputs=6
      settings: DisplayOption=none
  Mux1 : Mux  Inputs=6
  Product{2..5} (4 alike) : Product  InputSameDT=on  RndMeth=Zero  SaturateOnIntegerOverflow=on  OutDataTypeStr=Inherit: Same as first input
  Sum3 : Sum  Inputs=-+  InputSameDT=on  SaturateOnIntegerOverflow=on  OutDataTypeStr=Inherit: Same as first input
  Sum4 : Sum  Inputs=--  InputSameDT=on  SaturateOnIntegerOverflow=on  OutDataTypeStr=Inherit: Same as first input
  cos alpha : Fcn  Expr=cos(u[1])
  sin alpha : Fcn
  FbMb : Outport  VectorParamsAs1DForOutWhenUnconnected=off
  wires:
  Demux2/6 -> Mux1/6
  Demux2/5 -> Mux1/5
  Demux2/2 -> Mux1/2
  Demux2/4 -> Mux1/4
  cos alpha/1 -> Product2/1, Product5/1
  Demux2/1 -> Product2/2, Product4/2
  Product2/1 -> Sum3/1
  Product3/1 -> Sum3/2
  Sum3/1 -> Mux1/1
  sin alpha/1 -> Product3/1, Product4/1
  Demux2/3 -> Product3/2, Product5/2
  Product4/1 -> Sum4/1
  Product5/1 -> Sum4/2
  Sum4/1 -> Mux1/3
  alpha/1 -> sin alpha/1, cos alpha/1
  Mux1/1 -> FbMb/1
  FsMb/1 -> Demux2/1

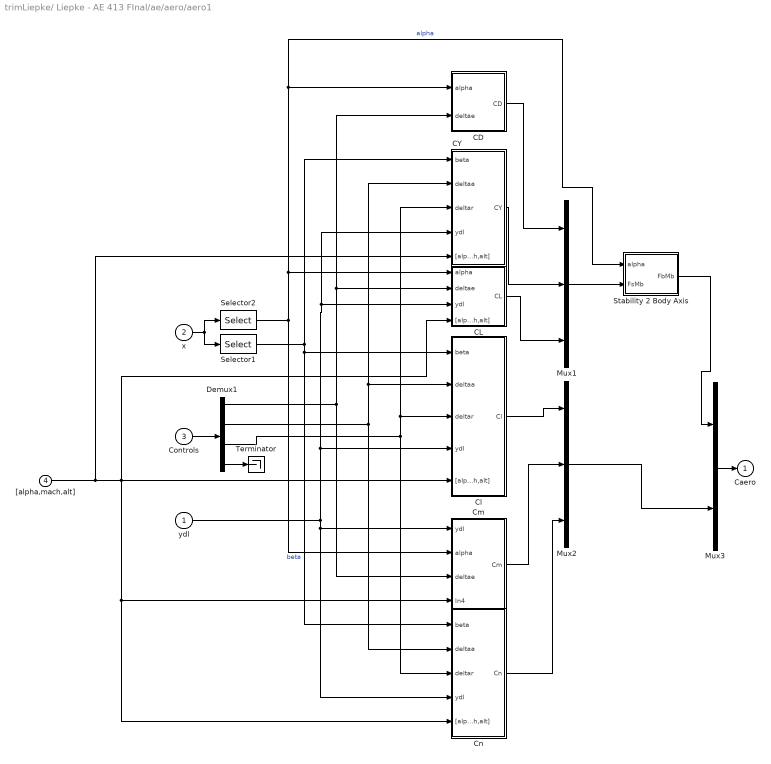
== system trimLiepke/ Liepke - AE 413 FInal/ae/aero/aero1 ==
  ydl : Inport
  x : Inport  Port=2
  Controls : Inport  Port=3
  "[alpha,mach,alt]" : Inport  Port=4
  CD : Subsystem
  CL : Subsystem
  CY : Subsystem
  Cl : Subsystem
  Cm : Subsystem
  Cn : Subsystem
  Demux1 : Demux
      settings: DisplayOption=none
  Mux1 : Mux  Inputs=3
  Mux2 : Mux  Inputs=3
  Mux3 : Mux  Inputs=2
  Selector1 : Selector  InputPortWidth=12  IndexOptions=Index vector (dialog)  Indices=[3]  OutputSizes=1
  Selector2 : Selector  InputPortWidth=12  IndexOptions=Index vector (dialog)  Indices=[2]  OutputSizes=1
  Stability 2 Body Axis : Subsystem
  Terminator : Terminator
  Caero : Outport  VectorParamsAs1DForOutWhenUnconnected=off
  wires:
  Demux1/3 -> CY/3(deltar), Cl/3(deltar), Cn/3(deltar)
  Demux1/2 -> CY/2(deltaa), Cl/2(deltaa), Cn/2(deltaa)
  Demux1/1 -> CD/2(deltae), CL/2(deltae), Cm/3(deltae)
  ydl/1 -> Cm/1(ydl), Cn/4(ydl), CY/4(ydl), CL/3(ydl), Cl/4(ydl)
  CD/1(CD) -> Mux1/1
  Mux1/1 -> Stability 2 Body Axis/2(FsMb)
  CY/1(CY) -> Mux1/2
  x/1 -> Selector2/1, Selector1/1
  Selector1/1 -> Cn/1(beta), Cl/1(beta), CY/1(beta)  "beta"
  Selector2/1 -> Cm/2(alpha), Stability 2 Body Axis/1(alpha), CD/1(alpha), CL/1(alpha)  "alpha"
  CL/1(CL) -> Mux1/3
  Controls/1 -> Demux1/1
  Demux1/4 -> Terminator/1
  Stability 2 Body Axis/1(FbMb) -> Mux3/1
  Cl/1(Cl) -> Mux2/1
  Cm/1(Cm) -> Mux2/2
  Cn/1(Cn) -> Mux2/3
  Mux3/1 -> Caero/1
  Mux2/1 -> Mux3/2
  "[alpha,mach,alt]"/1 -> CY/5("[alpha,mach,alt]"), CL/4("[alpha,mach,alt]"), Cl/5("[alpha,mach,alt]"), Cn/5("[alpha,mach,alt]"), Cm/4(In4)

== system trimLiepke/ Liepke - AE 413 FInal/ae/dl/0 ==

== system trimLiepke/ Liepke - AE 413 FInal/ae/fmdims/0 ==

== system trimLiepke/ Liepke - AE 413 FInal/eqm/ODE/0 ==

== system trimLiepke/ Liepke - AE 413 FInal/eqm/ODE/Eulerdot ==
  note: ueul=[x;Ftot;Mtot;yhlp]
  note: yeul=[psi dot; theta dot; phi dot]
  ueul : Inport
  0 : Subsystem
      mask Display: disp('EULERDOT\nM.O. Rauw, October 1997')
  Mux1 : Mux  Inputs=[29 1]
  Mux2 : Mux  Inputs=3
  phi dot : Fcn  Expr=u[4] + u[30]*u[26]
  psi dot : Fcn  Expr=(u[5]*u[28] + u[6]*u[29])/u[27]
  theta dot : Fcn  Expr=u[5]*u[29] - u[6]*u[28]
  yeul : Outport
  wires:
  ueul/1 -> theta dot/1, Mux1/1, psi dot/1
  psi dot/1 -> Mux2/1, Mux1/2
  theta dot/1 -> Mux2/2
  Mux2/1 -> yeul/1
  phi dot/1 -> Mux2/3
  Mux1/1 -> phi dot/1

== system trimLiepke/ Liepke - AE 413 FInal/eqm/ODE/Vabdot ==
  note: yVab=[V dot;alpha dot;beta dot]
  note: uVab=[x;Ftot;Mtot;yhlp]
  uVab : Inport
  0 : Subsystem
      mask Display: disp('VABDOT\nM.O. Rauw, October 1997')
  Mux2 : Mux  Inputs=3
  V dot : Fcn  Expr=(u[13]*u[19]*u[21]+u[14]*u[22]+u[15]*u[20]*u[21])/m
  alpha dot : Fcn  Expr=(-u[13]*u[20]+u[15]*u[19])/(m*u[1]*u[21]) - u[23]*(u[4]*u[19]+u[6]*u[20]) + u[5]
  beta dot : Fcn  Expr=(-u[13]*u[19]*u[22]+u[14]*u[21]-u[15]*u[20]*u[22])/(m*u[1]) + u[4]*u[20] - u[6]*u[19]
  yVab : Outport
  wires:
  beta dot/1 -> Mux2/3
  V dot/1 -> Mux2/1
  alpha dot/1 -> Mux2/2
  uVab/1 -> alpha dot/1, beta dot/1, V dot/1
  Mux2/1 -> yVab/1

== system trimLiepke/ Liepke - AE 413 FInal/eqm/ODE/pqrdot ==
  note: ytmp = [L; M; N; p^2; pq; pr; q^2; qr; r^2]
  note: upqr=[x;Ftot;Mtot;yhlp]
  note: ypqr=[p dot;q dot;r dot]
  note: ytmp
  note: Here: ypqr = GM2*ytmp
  note: [L M N]'
  note: [p q r]'
  upqr : Inport
  0 : Subsystem
      mask Display: disp('PQRDOT\nM.O. Rauw, October 1997')
  Demux : Demux  Outputs=[3 3 9 3 11]
      settings: DisplayOption=none
  Fcn : Fcn  Expr=u[1]^2
  Fcn1 : Fcn  Expr=u[1]*u[2]
  Fcn2 : Fcn  Expr=u[1]*u[3]
  Fcn3 : Fcn  Expr=u[2]^2
  Fcn4 : Fcn  Expr=u[2]*u[3]
  Fcn5 : Fcn  Expr=u[3]^2
  "GM2 " : Subsystem  mask(State Space){M=GM2}
      mask prompts: M "Matrix"
      mask Display: disp('Matrix\nGain')
  Mux : Mux  Inputs=[3 1 1 1 1 1 1]
  Terminator1 : Terminator
  Terminator2 : Terminator
  Terminator3 : Terminator
  ypqr : Outport
  wires:
  Mux/1 -> "GM2 "/1(In1)
  "GM2 "/1(Out1) -> ypqr/1
  Fcn5/1 -> Mux/7
  Fcn4/1 -> Mux/6
  Fcn3/1 -> Mux/5
  Fcn2/1 -> Mux/4
  Fcn1/1 -> Mux/3
  Fcn/1 -> Mux/2
  Demux/4 -> Mux/1
  Demux/2 -> Fcn3/1, Fcn5/1, Fcn4/1, Fcn2/1, Fcn/1, Fcn1/1
  Demux/3 -> Terminator1/1
  Demux/5 -> Terminator2/1
  Demux/1 -> Terminator3/1
  upqr/1 -> Demux/1

== system trimLiepke/ Liepke - AE 413 FInal/eqm/ODE/xyHdot ==
  note: uxyH=[x;Ftot;Mtot;yhlp]
  note: yxyH=[xe dot; ye dot; H dot]
  ybvel* : Inport
  uxYH : Inport  Port=2
  0 : Subsystem
      mask Display: disp('XYHDOT\nM.O. Rauw, October 1997')
  H dot : Fcn  Expr=u[30]*u[26] - (u[31]*u[28]+u[32]*u[29])*u[27]
  Mux2 : Mux  Inputs=[29 3]
  Mux3 : Mux  Inputs=2
  Mux4 : Mux  Inputs=[29 2]
  Mux5 : Mux  Inputs=3
  tmp1 : Fcn  Expr=u[30]*u[27] + (u[31]*u[28]+u[32]*u[29])*u[26]
  tmp2 : Fcn  Expr=u[31]*u[29] - u[32]*u[28]
  xe dot : Fcn  Expr=u[30]*u[25] - u[31]*u[24]
  ye dot : Fcn  Expr=u[30]*u[24] + u[31]*u[25]
  yxyH : Outport
  wires:
  uxYH/1 -> Mux2/1, Mux4/1
  ybvel*/1 -> Mux2/2
  Mux3/1 -> Mux4/2
  Mux2/1 -> tmp1/1, tmp2/1, H dot/1
  Mux4/1 -> xe dot/1, ye dot/1
  Mux5/1 -> yxyH/1
  ye dot/1 -> Mux5/2
  tmp2/1 -> Mux3/2
  xe dot/1 -> Mux5/1
  H dot/1 -> Mux5/3
  tmp1/1 -> Mux3/1

== system trimLiepke/ Liepke - AE 413 FInal/eqm/uvw/0 ==

== system trimLiepke/ Liepke - AE 413 FInal/eqm/xdotcorr/0 ==

== system trimLiepke/ Liepke - AE 413 FInal/out/accel/0 ==

== system trimLiepke/ Liepke - AE 413 FInal/out/fp/0 ==

== system trimLiepke/ Liepke - AE 413 FInal/out/uvwdot/0 ==

== system trimLiepke/ Liepke - AE 413 FInal/ae/aero/aero1/CD ==
  alpha : Inport
  deltae : Inport  Port=2
  CLa : Constant  Value=CD_alpha  SampleTime=-1
  CLa1 : Constant  Value=CD_0  SampleTime=-1
  CLde : Constant  Value=CD_de  SampleTime=-1
  Sum2 : Sum  Inputs=+++  InputSameDT=on  SaturateOnIntegerOverflow=on  OutDataTypeStr=Inherit: Same as first input
  n : Product  InputSameDT=on  SaturateOnIntegerOverflow=on  OutDataTypeStr=Inherit: Same as first input
  n1 : Product  InputSameDT=on  SaturateOnIntegerOverflow=on  OutDataTypeStr=Inherit: Same as first input
  CD : Outport  VectorParamsAs1DForOutWhenUnconnected=off
  wires:
  n/1 -> Sum2/2
  Sum2/1 -> CD/1
  n1/1 -> Sum2/1
  CLa1/1 -> Sum2/3
  alpha/1 -> n/1
  CLa/1 -> n/2
  deltae/1 -> n1/1
  CLde/1 -> n1/2

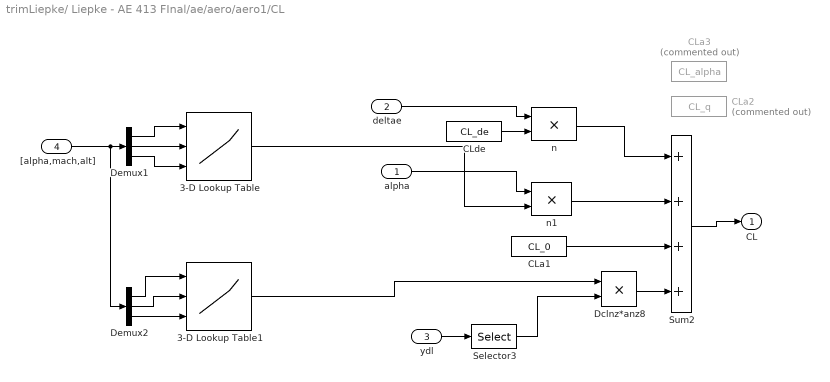
== system trimLiepke/ Liepke - AE 413 FInal/ae/aero/aero1/CL ==
  alpha : Inport
  deltae : Inport  Port=2
  ydl : Inport  Port=3
  "[alpha,mach,alt]" : Inport  Port=4
  3-D Lookup Table : Lookup_n-D  NumberOfTableDimensions=3  BreakpointsForDimension1=alpha_matrix  BreakpointsForDimension2=mach_matrix  BreakpointsForDimension3=alt_matrix  Table=cla_matrix  DiagnosticForOutOfRangeInput=Warning  InternalRulePriority=Speed  RndMeth=Simplest  InputSameDT=on
      settings: InputPortMap=u0,u1,u2
  3-D Lookup Table1 : Lookup_n-D  NumberOfTableDimensions=3  BreakpointsForDimension1=alpha_matrix  BreakpointsForDimension2=mach_matrix  BreakpointsForDimension3=alt_matrix  Table=clq_matrix  DiagnosticForOutOfRangeInput=Warning  InternalRulePriority=Speed  RndMeth=Simplest  InputSameDT=on
      settings: InputPortMap=u0,u1,u2
  CLa1 : Constant  Value=CL_0  SampleTime=-1
  CLa2 : Constant  Commented=on  Value=CL_q  SampleTime=-1
  CLa3 : Constant  Commented=on  Value=CL_alpha  SampleTime=-1
  CLde : Constant  Value=CL_de  SampleTime=-1
  Dclnz*anz8 : Product  InputSameDT=on  SaturateOnIntegerOverflow=on  OutDataTypeStr=Inherit: Same as first input
  Demux1 : Demux  Outputs=3
  Demux2 : Demux  Outputs=3
  Selector3 : Selector  InputPortWidth=3  IndexOptions=Index vector (dialog)  Indices=[2]  OutputSizes=1
  Sum2 : Sum  Inputs=++++  InputSameDT=on  SaturateOnIntegerOverflow=on  OutDataTypeStr=Inherit: Same as first input
  n : Product  InputSameDT=on  SaturateOnIntegerOverflow=on  OutDataTypeStr=Inherit: Same as first input
  n1 : Product  InputSameDT=on  SaturateOnIntegerOverflow=on  OutDataTypeStr=Inherit: Same as first input
  CL : Outport  VectorParamsAs1DForOutWhenUnconnected=off
  wires:
  CLa1/1 -> Sum2/3
  n/1 -> Sum2/1
  Sum2/1 -> CL/1
  n1/1 -> Sum2/2
  Dclnz*anz8/1 -> Sum2/4
  3-D Lookup Table1/1 -> Dclnz*anz8/1
  Selector3/1 -> Dclnz*anz8/2
  ydl/1 -> Selector3/1
  deltae/1 -> n/1
  CLde/1 -> n/2
  alpha/1 -> n1/1
  Demux1/1 -> 3-D Lookup Table/1
  Demux1/3 -> 3-D Lookup Table/3
  Demux1/2 -> 3-D Lookup Table/2
  "[alpha,mach,alt]"/1 -> Demux2/1, Demux1/1
  3-D Lookup Table/1 -> n1/2
  Demux2/2 -> 3-D Lookup Table1/2
  Demux2/3 -> 3-D Lookup Table1/3
  Demux2/1 -> 3-D Lookup Table1/1

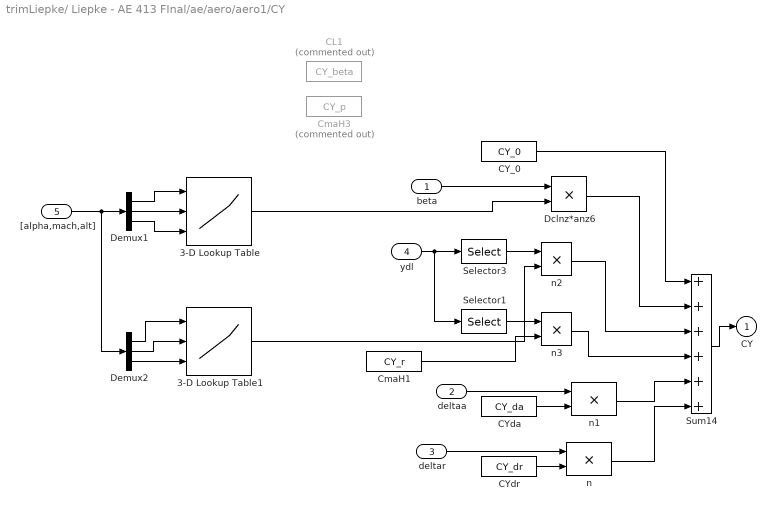
== system trimLiepke/ Liepke - AE 413 FInal/ae/aero/aero1/CY ==
  beta : Inport
  deltaa : Inport  Port=2
  deltar : Inport  Port=3
  ydl : Inport  Port=4
  "[alpha,mach,alt]" : Inport  Port=5
  3-D Lookup Table : Lookup_n-D  NumberOfTableDimensions=3  BreakpointsForDimension1=alpha_matrix  BreakpointsForDimension2=mach_matrix  BreakpointsForDimension3=alt_matrix  Table=cyb_matrix  InternalRulePriority=Speed  RndMeth=Simplest  InputSameDT=on
      settings: InputPortMap=u0,u1,u2
  3-D Lookup Table1 : Lookup_n-D  NumberOfTableDimensions=3  BreakpointsForDimension1=alpha_matrix  BreakpointsForDimension2=mach_matrix  BreakpointsForDimension3=alt_matrix  Table=cyp_matrix  InternalRulePriority=Speed  RndMeth=Simplest  InputSameDT=on
      settings: InputPortMap=u0,u1,u2
  CL1 : Constant  Commented=on  Value=CY_beta
  CY_0 : Constant  Value=CY_0
  CYda : Constant  Value=CY_da
  CYdr : Constant  Value=CY_dr
  CmaH1 : Constant  Value=CY_r
  CmaH3 : Constant  Commented=on  Value=CY_p
  Dclnz*anz6 : Product  InputSameDT=on  SaturateOnIntegerOverflow=on  OutDataTypeStr=Inherit: Same as first input
  Demux1 : Demux  Outputs=3
  Demux2 : Demux  Outputs=3
  Selector1 : Selector  InputPortWidth=3  IndexOptions=Index vector (dialog)  Indices=3  OutputSizes=1
  Selector3 : Selector  InputPortWidth=3  IndexOptions=Index vector (dialog)  Indices=1  OutputSizes=1
  Sum14 : Sum  Inputs=6  InputSameDT=on  SaturateOnIntegerOverflow=on  OutDataTypeStr=Inherit: Same as first input
  n{,1..3} (4 alike) : Product  InputSameDT=on  SaturateOnIntegerOverflow=on  OutDataTypeStr=Inherit: Same as first input
  CY : Outport  VectorParamsAs1DForOutWhenUnconnected=off
  wires:
  beta/1 -> Dclnz*anz6/1
  CYdr/1 -> n/2
  deltar/1 -> n/1
  CYda/1 -> n1/2
  deltaa/1 -> n1/1
  Selector3/1 -> n2/1
  ydl/1 -> Selector1/1, Selector3/1
  Selector1/1 -> n3/1
  Sum14/1 -> CY/1
  Dclnz*anz6/1 -> Sum14/2
  CY_0/1 -> Sum14/1
  n2/1 -> Sum14/3
  n3/1 -> Sum14/4
  n1/1 -> Sum14/5
  n/1 -> Sum14/6
  Demux1/1 -> 3-D Lookup Table/1
  Demux1/3 -> 3-D Lookup Table/3
  "[alpha,mach,alt]"/1 -> Demux2/1, Demux1/1
  Demux1/2 -> 3-D Lookup Table/2
  3-D Lookup Table/1 -> Dclnz*anz6/2
  Demux2/2 -> 3-D Lookup Table1/2
  Demux2/3 -> 3-D Lookup Table1/3
  Demux2/1 -> 3-D Lookup Table1/1
  3-D Lookup Table1/1 -> n2/2
  CmaH1/1 -> n3/2

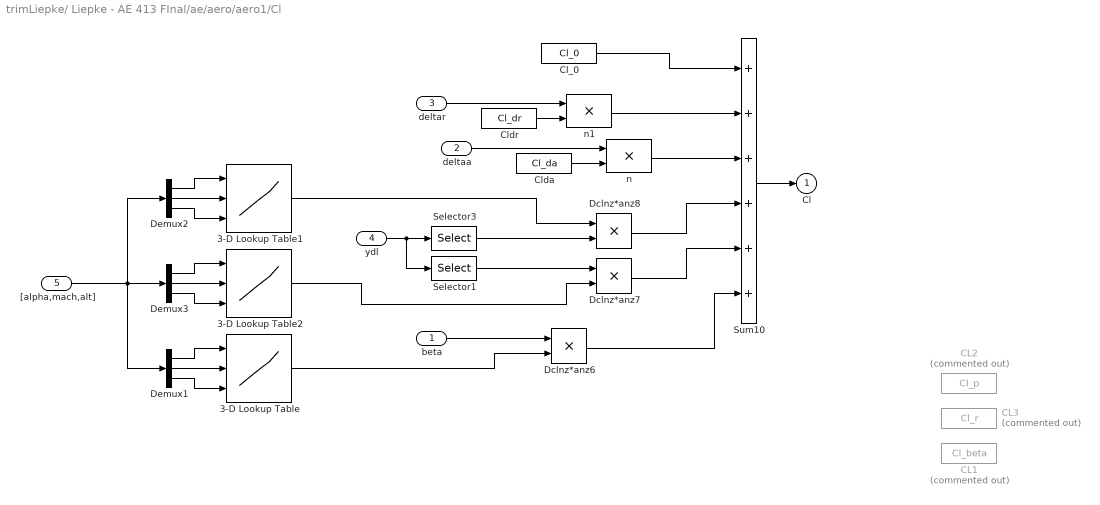
== system trimLiepke/ Liepke - AE 413 FInal/ae/aero/aero1/Cl ==
  beta : Inport
  deltaa : Inport  Port=2
  deltar : Inport  Port=3
  ydl : Inport  Port=4
  "[alpha,mach,alt]" : Inport  Port=5
  3-D Lookup Table : Lookup_n-D  NumberOfTableDimensions=3  BreakpointsForDimension1=alpha_matrix  BreakpointsForDimension2=mach_matrix  BreakpointsForDimension3=alt_matrix  Table=clb_matrix  InternalRulePriority=Speed  RndMeth=Simplest  InputSameDT=on
      settings: InputPortMap=u0,u1,u2
  3-D Lookup Table1 : Lookup_n-D  NumberOfTableDimensions=3  BreakpointsForDimension1=alpha_matrix  BreakpointsForDimension2=mach_matrix  BreakpointsForDimension3=alt_matrix  Table=clp_matrix  InternalRulePriority=Speed  RndMeth=Simplest  InputSameDT=on
      settings: InputPortMap=u0,u1,u2
  3-D Lookup Table2 : Lookup_n-D  NumberOfTableDimensions=3  BreakpointsForDimension1=alpha_matrix  BreakpointsForDimension2=mach_matrix  BreakpointsForDimension3=alt_matrix  Table=clr_matrix  InternalRulePriority=Speed  RndMeth=Simplest  InputSameDT=on
      settings: InputPortMap=u0,u1,u2
  CL1 : Constant  Commented=on  Value=Cl_beta
  CL2 : Constant  Commented=on  Value=Cl_p
  CL3 : Constant  Commented=on  Value=Cl_r
  Cl_0 : Constant  Value=Cl_0
  Clda : Constant  Value=Cl_da
  Cldr : Constant  Value=Cl_dr
  Dclnz*anz6 : Product  InputSameDT=on  SaturateOnIntegerOverflow=on  OutDataTypeStr=Inherit: Same as first input
  Dclnz*anz7 : Product  InputSameDT=on  SaturateOnIntegerOverflow=on  OutDataTypeStr=Inherit: Same as first input
  Dclnz*anz8 : Product  InputSameDT=on  SaturateOnIntegerOverflow=on  OutDataTypeStr=Inherit: Same as first input
  Demux1 : Demux  Outputs=3
  Demux2 : Demux  Outputs=3
  Demux3 : Demux  Outputs=3
  Selector1 : Selector  InputPortWidth=3  IndexOptions=Index vector (dialog)  Indices=[3]  OutputSizes=1
  Selector3 : Selector  InputPortWidth=3  IndexOptions=Index vector (dialog)  Indices=[1]  OutputSizes=1
  Sum10 : Sum  Inputs=++++++  InputSameDT=on  SaturateOnIntegerOverflow=on  OutDataTypeStr=Inherit: Same as first input
  n : Product  InputSameDT=on  SaturateOnIntegerOverflow=on  OutDataTypeStr=Inherit: Same as first input
  n1 : Product  InputSameDT=on  SaturateOnIntegerOverflow=on  OutDataTypeStr=Inherit: Same as first input
  Cl : Outport  VectorParamsAs1DForOutWhenUnconnected=off
  wires:
  n/1 -> Sum10/3
  Dclnz*anz7/1 -> Sum10/5
  Dclnz*anz8/1 -> Sum10/4
  Sum10/1 -> Cl/1
  3-D Lookup Table1/1 -> Dclnz*anz8/1
  Dclnz*anz6/1 -> Sum10/6
  ydl/1 -> Selector1/1, Selector3/1
  3-D Lookup Table2/1 -> Dclnz*anz7/2
  Selector1/1 -> Dclnz*anz7/1
  Selector3/1 -> Dclnz*anz8/2
  n1/1 -> Sum10/2
  beta/1 -> Dclnz*anz6/1
  deltaa/1 -> n/1
  Clda/1 -> n/2
  Cldr/1 -> n1/2
  deltar/1 -> n1/1
  Cl_0/1 -> Sum10/1
  Demux1/1 -> 3-D Lookup Table/1
  Demux1/3 -> 3-D Lookup Table/3
  Demux1/2 -> 3-D Lookup Table/2
  3-D Lookup Table/1 -> Dclnz*anz6/2
  "[alpha,mach,alt]"/1 -> Demux1/1, Demux2/1, Demux3/1
  Demux2/3 -> 3-D Lookup Table1/3
  Demux2/2 -> 3-D Lookup Table1/2
  Demux2/1 -> 3-D Lookup Table1/1
  Demux3/1 -> 3-D Lookup Table2/1
  Demux3/2 -> 3-D Lookup Table2/2
  Demux3/3 -> 3-D Lookup Table2/3
